simulink library "maskExprHandling_example_lib"  (R2018b)
settings: Solver=VariableStepAuto  StartTime=0.0  StopTime=10.0  RelTol=1e-3
undefined symbols (not defined in the file or in its folder): par_a
settings Model: Creator=jonas  LastModifiedBy=jonas

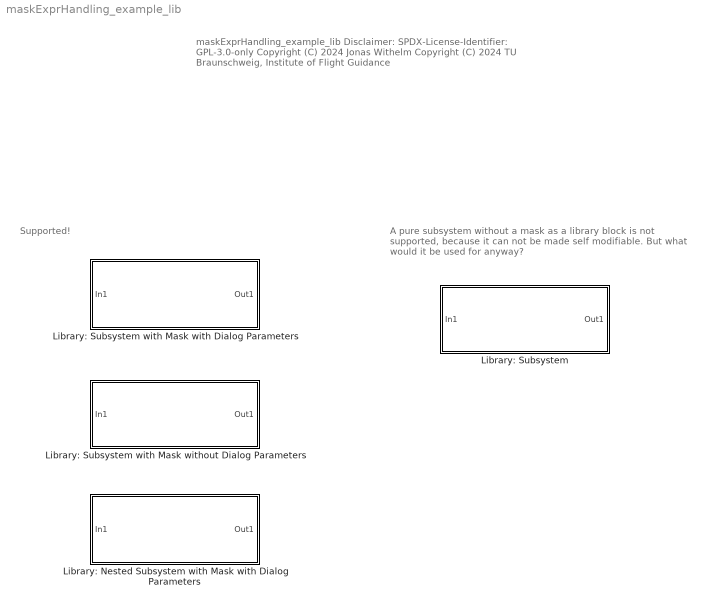
== system maskExprHandling_example_lib ==
  note: A pure subsystem without a mask as a library block is not supported, because it can not be made self modifiable.
      | But what would it be used for anyway?
  note: Supported!
  note: maskExprHandling_example_lib
      |
      | Disclaimer:
      | SPDX-License-Identifier: GPL-3.0-only
      |
      | Copyright (C) 2024 Jonas Withelm
      | Copyright (C) 2024 TU Braunschweig, Institute of Flight Guidance
  Library: Nested Subsystem with Mask with Dialog Parameters : Subsystem  mask{par_aa=2.*par_a, mask_expr_handling_config=default}
      mask prompts: par_aa "edit:"
      mask init:
      | maskExprHandling(gcbh, mask_expr_handling_config);
      mask TypeOptions mask_expr_handling_config: default | passthrough (tunable)
      mask DialogControl CodeGenerationSettings Prompt: Code Generation Settings
      mask DialogControl maskExprHandlingText Prompt: Mask expression handling
      mask DialogControl maskExprHandlingReadme Prompt: README
      mask DialogControl maskExprHandlingReadme Tooltip: https://github.com/iff-gsc/m-Utils/tree/main/simulink/mask_expression_handling/README.md
      mask DialogControl maskExprHandlingReadme Callback: web('https://github.com/iff-gsc/m-Utils/tree/main/simulink/mask_expression_handling/README.md','-browser')
  Library: Subsystem : Subsystem
  Library: Subsystem with Mask with Dialog Parameters : Subsystem  mask{par_aa=2.*par_a, mask_expr_handling_config=default}
      mask prompts: par_aa "edit:"
      mask init:
      | maskExprHandling(gcbh, mask_expr_handling_config);
      mask TypeOptions mask_expr_handling_config: default | passthrough (tunable)
      mask DialogControl CodeGenerationSettings Prompt: Code Generation Settings
      mask DialogControl maskExprHandlingText Prompt: Mask expression handling
      mask DialogControl maskExprHandlingReadme Prompt: README
      mask DialogControl maskExprHandlingReadme Tooltip: https://github.com/iff-gsc/m-Utils/tree/main/simulink/mask_expression_handling/README.md
      mask DialogControl maskExprHandlingReadme Callback: web('https://github.com/iff-gsc/m-Utils/tree/main/simulink/mask_expression_handling/README.md','-browser')
  Library: Subsystem with Mask without Dialog Parameters : Subsystem

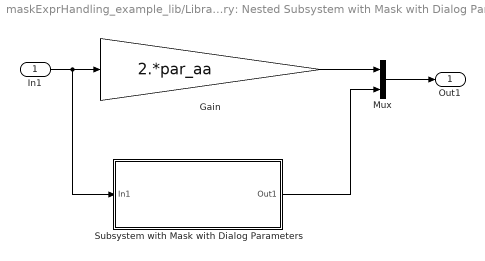
== system maskExprHandling_example_lib/Library: Nested Subsystem with Mask with Dialog Parameters ==
  In1 : Inport
  Gain : Gain  Gain=2.*par_aa
  Mux : Mux  Inputs=2
  Subsystem with Mask with Dialog Parameters : Subsystem  mask{par_aaa=2.*par_aa, mask_expr_handling_config=default}
      mask prompts: par_aaa "edit:"
      mask init:
      | maskExprHandling(gcbh, mask_expr_handling_config);
      mask TypeOptions mask_expr_handling_config: default | passthrough (tunable)
      mask DialogControl CodeGenerationSettings Prompt: Code Generation Settings
      mask DialogControl maskExprHandlingText Prompt: Mask expression handling
      mask DialogControl maskExprHandlingReadme Prompt: README
      mask DialogControl maskExprHandlingReadme Tooltip: https://github.com/iff-gsc/m-Utils/tree/main/simulink/mask_expression_handling/README.md
      mask DialogControl maskExprHandlingReadme Callback: web('https://github.com/iff-gsc/m-Utils/tree/main/simulink/mask_expression_handling/README.md','-browser')
  Out1 : Outport
  wires:
  Gain/1 -> Mux/1
  In1/1 -> Gain/1, Subsystem with Mask with Dialog Parameters/1(In1)
  Subsystem with Mask with Dialog Parameters/1(Out1) -> Mux/2
  Mux/1 -> Out1/1

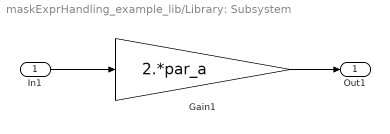
== system maskExprHandling_example_lib/Library: Subsystem ==
  In1 : Inport
  Gain1 : Gain  Gain=2.*par_a
  Out1 : Outport
  wires:
  Gain1/1 -> Out1/1
  In1/1 -> Gain1/1

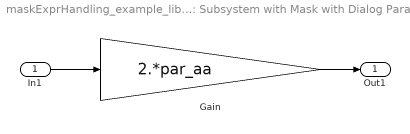
== system maskExprHandling_example_lib/Library: Subsystem with Mask with Dialog Parameters ==
  In1 : Inport
  Gain : Gain  Gain=2.*par_aa
  Out1 : Outport
  wires:
  In1/1 -> Gain/1
  Gain/1 -> Out1/1

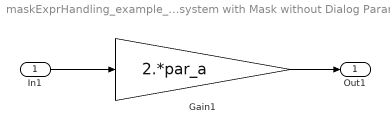
== system maskExprHandling_example_lib/Library: Subsystem with Mask without Dialog Parameters ==
  In1 : Inport
  Gain1 : Gain  Gain=2.*par_a
  Out1 : Outport
  wires:
  Gain1/1 -> Out1/1
  In1/1 -> Gain1/1

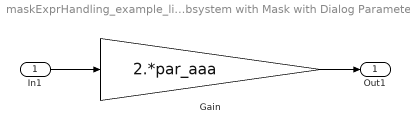
== system maskExprHandling_example_lib/Library: Nested Subsystem with Mask with Dialog Parameters/Subsystem with Mask with Dialog Parameters ==
  In1 : Inport
  Gain : Gain  Gain=2.*par_aaa
  Out1 : Outport
  wires:
  Gain/1 -> Out1/1
  In1/1 -> Gain/1
